simulink model "oscilloscope"  (Simulink 2.09)
settings: Solver=ode4  StartTime=0  StopTime=999999999999999999999999  RelTol=1e-3  AbsTol=1e-6
libraries: simulink x2
settings Model: ConsistencyChecking=off  RTWTemplateMakefile=grt_vc.tmf

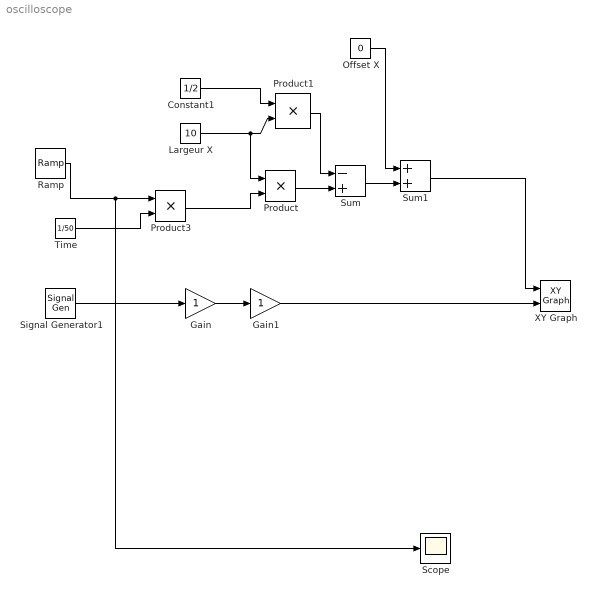
== system oscilloscope ==
  Constant1 : Constant  Value=1/2
  Gain : Gain  Gain=1
  Gain1 : Gain  Gain=1
  Largeur X : Constant  Value=10
  Offset X : Constant  Value=0
  Product : Product  Inputs=2
  Product1 : Product  Inputs=2
  Product3 : Product  Inputs=2
  Ramp : simulink/Sources/Ramp  slope=1  start=0  X0=0
  Scope : Scope
      settings: TickLabels=on  TimeRange=auto  YMin=-5  YMax=5  SaveToWorkspace=off  SaveName=ScopeData
  Signal Generator1 : SignalGenerator  WaveForm=sine  Amplitude=3  Frequency=1  Units=Hertz
  Sum : Sum  Inputs=-+
  Sum1 : Sum  Inputs=++
  Time : Constant  Value=1/50
  XY Graph : simulink/Sinks/XY Graph  xmin=-5  xmax=5  ymin=-5  ymax=5  st=-1
  wires:
  Gain/1 -> Gain1/1
  Ramp/1 -> Scope/1, Product3/1
  Signal Generator1/1 -> Gain/1
  Time/1 -> Product3/2
  Product3/1 -> Product/2
  Gain1/1 -> XY Graph/2
  Constant1/1 -> Product1/1
  Largeur X/1 -> Product1/2, Product/1
  Offset X/1 -> Sum1/1
  Sum1/1 -> XY Graph/1
  Sum/1 -> Sum1/2
  Product1/1 -> Sum/1
  Product/1 -> Sum/2
